simulink model "Bull_Cow"  (R2022b)
settings: Solver=FixedStepDiscrete  StartTime=0.0  StopTime=100  RelTol=1e-3
InitFcn:
  | mbd_s32k_consistency_checks(bdroot(gcs));
undefined symbols (not defined in the file): LQFP
libraries: mbd_s32k1xx_ec_toolbox x7, simulink x1, aerolibanimutils x1
settings Model: Creator=termi  LastModifiedBy=termi
settings DataIOCC: ExternalInput=off  InitialState=off  SaveOutput=off  SignalLogging=off  SaveTime=off
settings OptimizationCC: DefaultParameterBehavior=Inlined  EnhancedBackFolding=on  PassReuseOutputArgsAs=Individual arguments  ZeroExternalMemoryAtStartup=off  ZeroInternalMemoryAtStartup=off  OptimizeBlockOrder=speed  DifferentSizesBufferReuse=on  OptimizationCustomize=off  EfficientTunableParamExpr=on
settings DebuggingCC: InheritedTsInSrcMsg=none  SingleTaskRateTransMsg=error  ParameterTunabilityLossMsg=error  UnconnectedInputMsg=error  UnconnectedOutputMsg=error  UnconnectedLineMsg=error  UnknownTsInhSupMsg=error
settings HardwareCC: ProdBitPerPointer=32  ProdBitPerSizeT=32  ProdBitPerPtrDiffT=32  ProdLargestAtomicInteger=Long  ProdLargestAtomicFloat=Double  ProdWordSize=32  ProdHWDeviceType=ARM Compatible->ARM Cortex
settings SFSimCC: MATLABDynamicMemAlloc=off
settings RTWCC: Description=Model Based Design Toolbox S32K1xx Code Generation Target  SystemTargetFile=mbd_s32k.tlc  MakeCommand=mbd_s32k_make_rtw COPY_MDLREF_INCLUDES=0  TemplateMakefile=mbd_s32k.tmf
settings CodeAppCC: ForceParamTrailComments=on  IgnoreCustomStorageClasses=off  OperatorAnnotations=on  SimulinkDataObjDesc=on  SFDataObjDesc=on  InsertBlockDesc=on
settings STFCustomTargetCC: TargetLangStandard=C99 (ISO)  MultiwordLength=256  CombineOutputUpdateFcns=on  ERTCustomFileBanners=on  SupportContinuousTime=off  SupportNonInlinedSFcns=off  RemoveResetFunc=on  MATLABClassNameForMDSCustomization=Simulink.SoftwareTarget.ERTCustomization  SystemTargetFile=mbd_s32k.tlc
settings ERTTargetCC: TargetLangStandard=C99 (ISO)  ParMdlRefBuildCompliant=off  CompOptLevelCompliant=off  ConcurrentExecutionCompliant=off  ModelStepFunctionPrototypeControlCompliant=off  CPPClassGenCompliant=off  UseToolchainInfoCompliant=off  InlinedParameterPlacement=NonHierarchical  ERTSrcFileBannerTemplate=mbd_ert_code_template.cgt  ERTHdrFileBannerTemplate=mbd_ert_code_template.cgt  ERTDataSrcFileTemplate=mbd_ert_code_template.cgt  ERTDataHdrFileTemplate=mbd_ert_code_template.cgt  ERTCustomFileTemplate=example_file_process.tlc

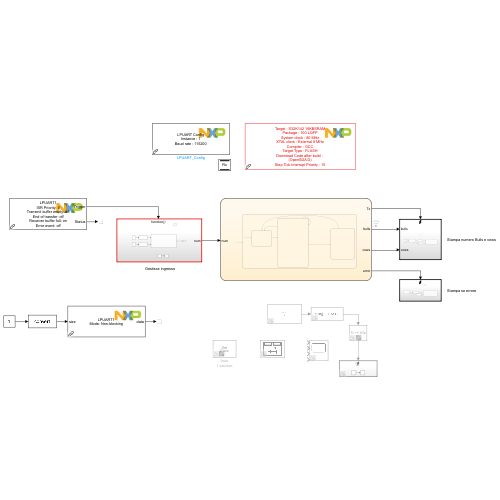
[thumbnail: Simulink's stored preview of the top-level diagram]
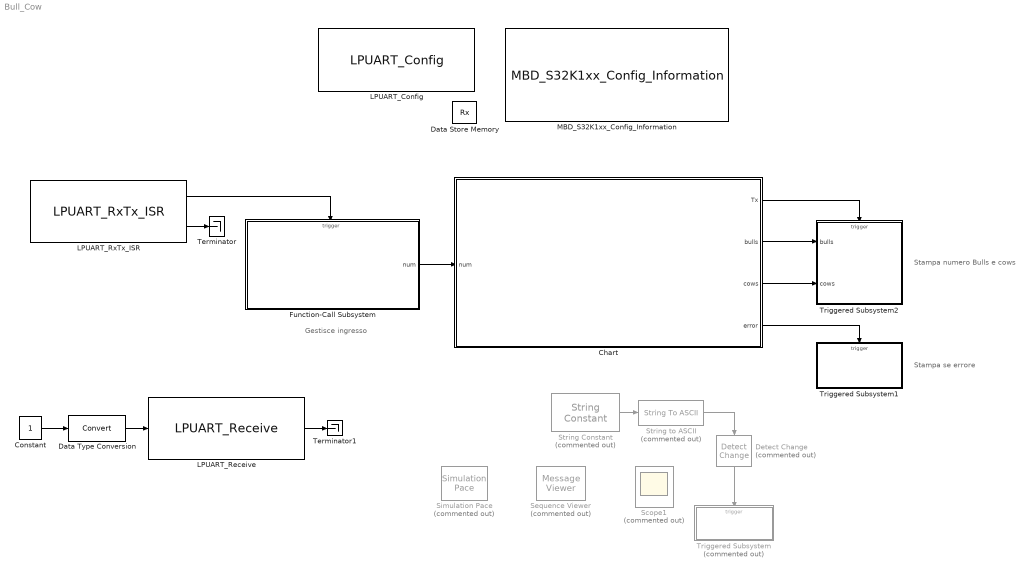
== system Bull_Cow ==
  note: Gestisce ingresso
  note: Stampa se errore
  note: Stampa numero Bulls e cows
  Chart : Stateflow chart  TreatAsAtomicUnit=on
  Constant : Constant
  Data Store Memory : DataStoreMemory  DataStoreName=Rx  WriteAfterWriteMsg=warning  ShowAdditionalParam=off  OutDataTypeStr=uint8
  Data Type Conversion : DataTypeConversion  SaturateOnIntegerOverflow=off  RndMeth=Floor
  Detect Change : simulink/Logic and Bit Operations/Detect Change  Commented=on  vinit=0  OutDataTypeStr=uint8
  Function-Call Subsystem : Subsystem  TreatAsAtomicUnit=on
  LPUART_Config : mbd_s32k1xx_ec_toolbox/Communication Blocks/UART Blocks/LPUART_Config  Priority=1  instance=1  baudrate=115200  custom_baudrate=1000000  databits=8  parity=None  sbns=1  bothedge=rising edge  rxinv=off  txinv=off  show_adv_opts=on  brk13=10 - 13 bit times  lbkde=10 - 13 bit times  rx=PTC6: [LPUART1_RX | Receive]  tx=PTC7: [LPUART1_TX | Transmit]
  LPUART_Receive : mbd_s32k1xx_ec_toolbox/Communication Blocks/UART Blocks/LPUART_Receive  Priority=2  instance=1  receive_mode=Non-blocking  timeout=500
  LPUART_RxTx_ISR : mbd_s32k1xx_ec_toolbox/Communication Blocks/UART Blocks/LPUART_RxTx_ISR  instance=1  prio=0  tie=off  tcie=off  rie=on  ilie=off
  MBD_S32K1xx_Config_Information : mbd_s32k1xx_ec_toolbox/MBD_S32K1xx_Config_Information  Priority=1  mbdt_ver=0  disp_str=|  config_params=[]  mcu_target_name=S32K142  mcu_target_package=100-LQFP  mcu_target_sram_size=16KB  mcu_system_clock_freq=80  mcu_xtal_freq=External 8  mcu_steptick_timer=LPIT Channel 0  mcu_steptick_prio=15  ds_import_enable=on  target_compiler=GCC  target_memory=FLASH  gcc_target_compile_opts=-mthumb -mfloat-abi=hard -mfpu=fpv4-sp-d16 -O1 -g -gstrict-dwarf  gcc_target_assemble_opts=-mthumb -mfloat-abi=hard -mfpu=fpv4-sp-d16 -g  gcc_target_link_opts=-mthumb -mfloat-abi=hard -mfpu=fpv4-sp-d16  gcc_target_default_lcf=on  gcc_target_user_lcf=S32K142_16_flash.ld  ghs_target_compile_opts=-cpu=cortexm4f -thumb -fpu=vfpv4_d16 -fsingle -Ogeneral -Wundef -Wimplicit-int -Wshadow -Wtrigraphs --no_commons --gnu_asm -gnu99 -gdwarf-2 -G  ghs_target_assemble_opts=-cpu=cortexm4f -fpu=vfpv4_d16  ghs_target_link_opts=-cpu=cortexm4f -thumb -fpu=vfpv4_d16  ghs_target_default_lcf=on  ghs_target_user_lcf=S32K142_16_flash.ld  iar_target_compile_opts=--cpu=Cortex-M4F --thumb --fpu=VFPv4_sp -Ol -e --debug --dlib_config normal  iar_target_assemble_opts=--cpu Cortex-M4F --thumb --fpu VFPv4_sp  iar_target_link_opts=--no_exceptions --vfe --inline  iar_target_default_lcf=on  iar_target_user_lcf=S32K142_16_flash.icf  pil_download_enable=off  rbl_download_enable=on  rbl_start_delay=5000  rbl_download_interface=OpenSDA  rbl_restart_request=off  rbl_com_port=Custom  rbl_com_port_custom=COM3  pil_download_rate=115200  pil_download_rate_custom=115200  pil_opensda_drive=Custom  pil_opensda_drive_custom=D  jtag_interface=OpenSDA Embedded Debug  jlink_default_path=on  jlink_user_path=C:\Program Files\SEGGER\JLink\  pil_uart_instance=1  pil_uart_rx=PTC6: [LPUART1_RX | Receive]  pil_uart_tx=PTC7: [LPUART1_TX | Transmit]  FTM_PWM_PcrCheckEnDis=on  FTM_Input_Edge_Inputs_PcrCheckEnDis=on  FTM_Dual_Edge_Inputs_PcrCheckEnDis=on  FTM_Quadrature_Inputs_PcrCheckEnDis=on  FTM_Hall_Sensor_Inputs_PcrCheckEnDis=on  LPTMR_PcrCheckEnDis=on  PIT_PcrCheckEnDis=on  RTC_PcrCheckEnDis=on  FlexCAN_PcrCheckEnDis=on  LIN_PcrCheckEnDis=on  FlexIO_PcrCheckEnDis=on  LPI2C_PcrCheckEnDis=on  LPSPI_PcrCheckEnDis=on  LPUART_PcrCheckEnDis=on  CMP_PcrCheckEnDis=on  GPIO_OutputPcrCheckEnDis=on  GPIO_InputPcrCheckEnDis=on  SBC_PcrCheckEnDis=on  BMS_PcrCheckEnDis=on  AMMCLIB_PcrCheckEnDis=on  FM_PcrCheckEnDis=on  Profile_PcrCheckEnDis=on  ConfigParams_PcrCheckEnDis=on  ModelRef_PcrCheckEnDis=on  PDB0_PcrCheckEnDis=on  CSEc_PcrCheckEnDis=on  eDMA_PcrCheckEnDis=on  FLASH_PcrCheckEnDis=on  ADC_PcrCheckEnDis=on  WDOG_PcrCheckEnDis=on
      | Target : S32K144-64KB_SRAM
      | Package : 100-pin
      | System clock : 80 MHz
      | XTAL clock : External 8 MHz
      | Compiler : IAR
      | Target Type : FLASH
      | Download Code after build : off
      | Step Tick Interrupt Priority : 15
  Scope1 : Scope  Commented=on  NumInputPorts=4
  Sequence Viewer : MessageViewer  Commented=on
  Simulation Pace : aerolibanimutils/Simulation Pace  Commented=on  SimulationPace=1  SleepMode=Auto  OutputPaceError=off  SampleTime=1/10
  String Constant : StringConstant  Commented=on  String="\";\""
  String to ASCII : StringToASCII  Commented=on  OutputVectorSize=1
  Terminator : Terminator
  Terminator1 : Terminator
  Triggered Subsystem : Subsystem  Commented=on  TreatAsAtomicUnit=on
  Triggered Subsystem1 : Subsystem  TreatAsAtomicUnit=on
  Triggered Subsystem2 : Subsystem  TreatAsAtomicUnit=on
  wires:
  String to ASCII/1 -> Detect Change/1
  Detect Change/1 -> Triggered Subsystem/Trigger
  String Constant/1 -> String to ASCII/1
  Data Type Conversion/1 -> LPUART_Receive/1
  LPUART_Receive/1 -> Terminator1/1
  Constant/1 -> Data Type Conversion/1
  LPUART_RxTx_ISR/2 -> Terminator/1
  LPUART_RxTx_ISR/1 -> Function-Call Subsystem/Trigger
  Chart/2(bulls) -> Triggered Subsystem2/1(bulls)
  Chart/3(cows) -> Triggered Subsystem2/2(cows)
  Chart/4(error) -> Triggered Subsystem1/Trigger
  Chart/1(Tx) -> Triggered Subsystem2/Trigger
  Function-Call Subsystem/1(num) -> Chart/1(num)

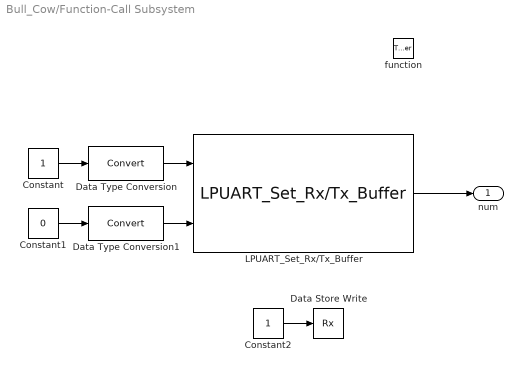
== system Bull_Cow/Function-Call Subsystem ==
  function : TriggerPort  TriggerType=function-call  VariantControl=(inherit)
  Constant : Constant
  Constant1 : Constant  Value=0
  Constant2 : Constant  OutDataTypeStr=uint8
  Data Store Write : DataStoreWrite  DataStoreName=Rx  IndexOptions=Index vector (dialog)  Indices=1  OutputSizes=1
  Data Type Conversion : DataTypeConversion  SaturateOnIntegerOverflow=off  RndMeth=Floor
  Data Type Conversion1 : DataTypeConversion  SaturateOnIntegerOverflow=off  RndMeth=Floor
  LPUART_Set_Rx/Tx_Buffer : mbd_s32k1xx_ec_toolbox/Communication Blocks/UART Blocks/LPUART_Set_Rx//Tx_Buffer  Priority=2  instance=1  buffer=Rx
  num : Outport
  wires:
  Constant/1 -> Data Type Conversion/1
  Data Type Conversion/1 -> LPUART_Set_Rx/Tx_Buffer/1
  Constant1/1 -> Data Type Conversion1/1
  Data Type Conversion1/1 -> LPUART_Set_Rx/Tx_Buffer/2
  LPUART_Set_Rx/Tx_Buffer/1 -> num/1
  Constant2/1 -> Data Store Write/1

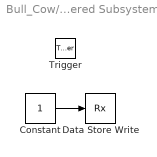
== system Bull_Cow/Triggered Subsystem ==
  Trigger : TriggerPort  VariantControl=(inherit)
  Constant : Constant  OutDataTypeStr=uint8
  Data Store Write : DataStoreWrite  DataStoreName=Rx  IndexOptions=Index vector (dialog)  Indices=1  OutputSizes=1
  wires:
  Constant/1 -> Data Store Write/1

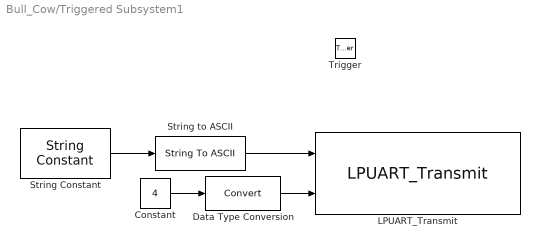
== system Bull_Cow/Triggered Subsystem1 ==
  Trigger : TriggerPort  VariantControl=(inherit)
  Constant : Constant  Value=4
  Data Type Conversion : DataTypeConversion  SaturateOnIntegerOverflow=off  RndMeth=Floor
  LPUART_Transmit : mbd_s32k1xx_ec_toolbox/Communication Blocks/UART Blocks/LPUART_Transmit  instance=1  transmit_mode=Non-blocking  timeout=500  number=on
  String Constant : StringConstant  String="\"ERRO\""
  String to ASCII : StringToASCII  OutputVectorSize=4
  wires:
  String Constant/1 -> String to ASCII/1
  String to ASCII/1 -> LPUART_Transmit/1
  Constant/1 -> Data Type Conversion/1
  Data Type Conversion/1 -> LPUART_Transmit/2

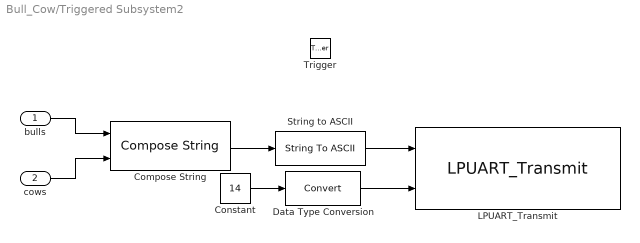
== system Bull_Cow/Triggered Subsystem2 ==
  bulls : Inport
  cows : Inport  Port=2
  Trigger : TriggerPort  VariantControl=(inherit)
  Compose String : ComposeString  Format="\"%u Bulls %u Cows\""
  Constant : Constant  Value=14
  Data Type Conversion : DataTypeConversion  SaturateOnIntegerOverflow=off  RndMeth=Floor
  LPUART_Transmit : mbd_s32k1xx_ec_toolbox/Communication Blocks/UART Blocks/LPUART_Transmit  instance=1  transmit_mode=Non-blocking  timeout=500  number=on
  String to ASCII : StringToASCII  OutputVectorSize=14
  wires:
  bulls/1 -> Compose String/1
  String to ASCII/1 -> LPUART_Transmit/1
  Constant/1 -> Data Type Conversion/1
  cows/1 -> Compose String/2
  Data Type Conversion/1 -> LPUART_Transmit/2
  Compose String/1 -> String to ASCII/1

== stateflow chart Bull_Cow/Chart ==
  note: Master_num const = [0;4;1;2]
      | str_lenght const = 5
  state Declarations
    en:
    str_lenght ;
    master_num;
    k = 1;
    error = 0;
    bulls = 0;
    cows = 0;
    state Error_check
      en:
      %Reset variabili
      bulls = 0;
      cows = 0;
      Tx = 0;
      Rx = 0;
      %Controllo se ingresso valido
      if (( num >= '0' && num <= '9') || num == ';')
      %Check ripetizioni
      for i = 1 : k
      if (str ( i ) == num)
      error  = 1;
      end;
      end;
      %Check " ; "
      if(k == str_lenght && num ~= ';' )
      error = 1;
      end
      %Check " ; " non in fondo
      if (k < str_lenght && num == ';')
      error = 1;
      end
      %Riempio vettore da checkare
      if (error == 0)
      str( k ) = num;
      k = k + 1;
      end;
      else
      error = 1;
      end;
    state Bulls_cows_check
      en:
      %Scorro i due vettori per compararli
      for i = 1 : (str_lenght -1)
      for j = 1 : (str_lenght -1)
      if (str( i ) == master_num ( j ))
      %Check bulls
      if( i == j)
      bulls = bulls + 1;
      %Check cows
      else
      cows = cows +1;
      end
      end
      end
      end
      exit:
      %Segnale trasmissione uscita
      Tx = 1;
    state Wait
      en:
      error = 0;
      k = 1;
      for i = 1 : (str_lenght)
      str ( i ) = 0;
      end
    note: Attendo per l'arrivo del primo carattere
        | da UART
    Bulls_cows_check -> Wait
    Error_check -> Error_check [order 3] : [Rx ==1 && error == 0]
    Error_check -> Wait [order 1] : [error == 1]
    Wait -> Error_check : [Rx==1]
    (default) -> Wait
    Error_check -> Bulls_cows_check [order 2] : [k == str_lenght + 1 && error == 0]
  (default) -> Declarations
  data: Tx output; num input uint8; bulls output uint8; cows output uint8; master_num constant uint8 size=4 =uint8(['0'; '4'; '1'; '2']); str_lenght constant uint8 =5; i local uint8; error output uint8; str local uint8 size=5 =uint8 ([0; 0; 0; 0; 0]); j local uint8; k local uint8; Rx data_store_memory
